simulink model "invariant1"  (Simulink 7.3)
settings: Solver=ode45  StartTime=0.0  StopTime=5  RelTol=1e-3
settings Model: Creator=Sainquake  LastModifiedBy=Sainquake Notebook

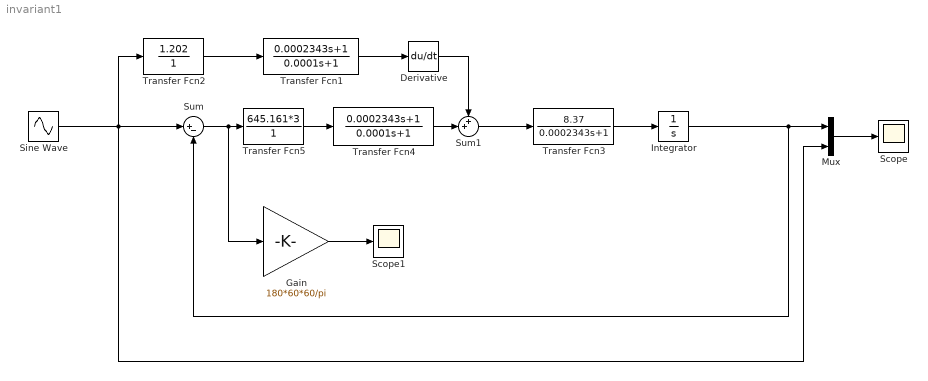
== system invariant1 ==
  Derivative : Derivative
  Gain : Gain  Gain=180*60*60/pi  ParameterDataType=fixdt(1, 16)  ParameterScaling=2^0  OutDataType=fixdt(1, 16)  OutScaling=2^0
  Integrator : Integrator
  Mux : Mux  Inputs=2
  Scope : Scope
      settings: MaxDataPoints=500000
  Scope1 : Scope
      settings: YMin=-0.45  YMax=0.25  MaxDataPoints=500000
  Sine Wave : Sin  Amplitude=2/180*pi  Bias=0  Frequency=1  Phase=0  Samples=10  SampleTime=0  Offset=0
  Sum : Sum  Inputs=|+-  OutDataType=fixdt(1, 16)  OutScaling=2^0
  Sum1 : Sum  Inputs=++|  OutDataType=fixdt(1, 16)  OutScaling=2^0
  Transfer Fcn1 : TransferFcn  Numerator=[0.0002343 1]  Denominator=[0.0001 1]
  Transfer Fcn2 : TransferFcn  Numerator=1.202  Denominator=1
  Transfer Fcn3 : TransferFcn  Numerator=[8.37]  Denominator=[0.0002343 1]
  Transfer Fcn4 : TransferFcn  Numerator=[0.0002343 1]  Denominator=[0.0001 1]
  Transfer Fcn5 : TransferFcn  Numerator=645.161*3  Denominator=1
  wires:
  Integrator/1 -> Sum/2, Mux/1
  Sine Wave/1 -> Sum/1, Transfer Fcn2/1, Mux/2
  Sum1/1 -> Transfer Fcn3/1
  Transfer Fcn2/1 -> Transfer Fcn1/1
  Sum/1 -> Transfer Fcn5/1, Gain/1
  Transfer Fcn1/1 -> Derivative/1
  Transfer Fcn3/1 -> Integrator/1
  Derivative/1 -> Sum1/1
  Transfer Fcn4/1 -> Sum1/2
  Transfer Fcn5/1 -> Transfer Fcn4/1
  Mux/1 -> Scope/1
  Gain/1 -> Scope1/1
